simulink model "hw3_sim"  (R2022a)
settings: Solver=VariableStepAuto  StartTime=0.0  StopTime=20  RelTol=1e-3
values from neighbouring files (symbols this model uses):
  ctrl = c*K    [h3.m]
  x0 = [10 0 10 0]'    [h3.m]
settings Model: Creator=voidjocker  LastModifiedBy=voidjocker

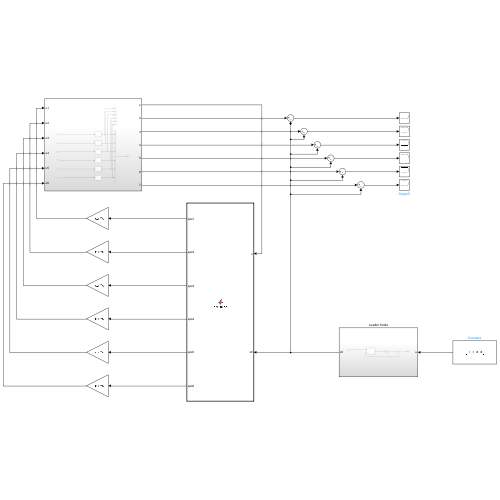
[thumbnail: Simulink's stored preview of the top-level diagram]
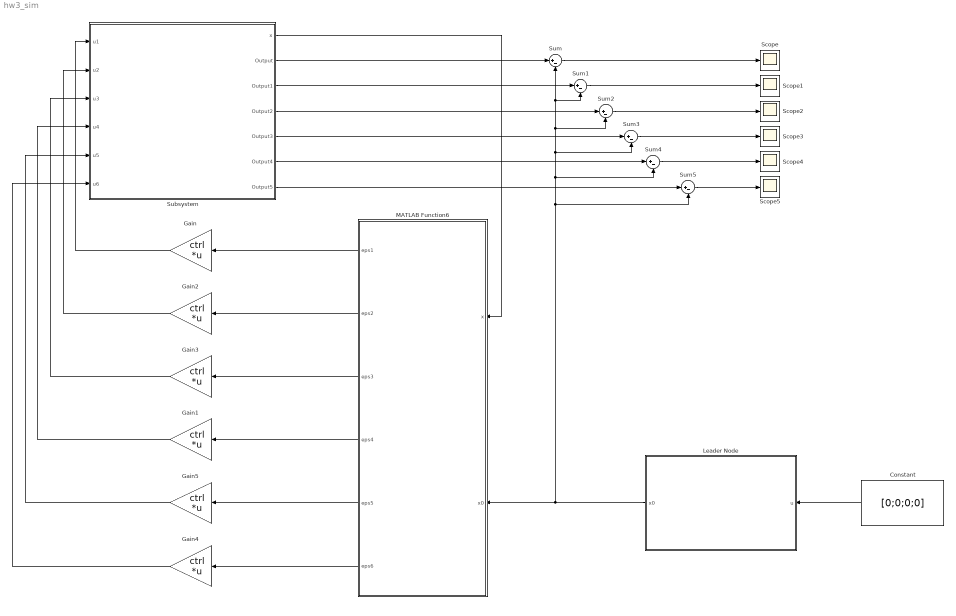
== system hw3_sim ==
  Constant : Constant  Value=[0;0;0;0]
  Gain{,1..5} (6 alike) : Gain  Gain=ctrl  Multiplication=Matrix(K*u)
  Leader Node : Subsystem
  MATLAB Function6 : MATLAB Function  TreatAsAtomicUnit=on
  Scope{,1..5} (6 alike) : Scope
  Subsystem : Subsystem
  Sum{,1..5} (6 alike) : Sum  Inputs=|+-
  wires:
  Constant/1 -> Leader Node/1(u)
  Leader Node/1(x0) -> Sum5/2, Sum4/2, Sum3/2, Sum2/2, Sum1/2, Sum/2, MATLAB Function6/2(x0)
  Subsystem/1(x) -> MATLAB Function6/1(x)
  Gain/1 -> Subsystem/1(u1)
  MATLAB Function6/1(eps1) -> Gain/1
  MATLAB Function6/2(eps2) -> Gain2/1
  MATLAB Function6/5(eps5) -> Gain5/1
  MATLAB Function6/4(eps4) -> Gain1/1
  MATLAB Function6/3(eps3) -> Gain3/1
  MATLAB Function6/6(eps6) -> Gain4/1
  Gain2/1 -> Subsystem/2(u2)
  Gain3/1 -> Subsystem/3(u3)
  Gain1/1 -> Subsystem/4(u4)
  Gain5/1 -> Subsystem/5(u5)
  Gain4/1 -> Subsystem/6(u6)
  Subsystem/2(Output) -> Sum/1
  Sum/1 -> Scope/1
  Subsystem/3(Output1) -> Sum1/1
  Subsystem/4(Output2) -> Sum2/1
  Sum2/1 -> Scope2/1
  Sum1/1 -> Scope1/1
  Sum3/1 -> Scope3/1
  Subsystem/5(Output3) -> Sum3/1
  Subsystem/6(Output4) -> Sum4/1
  Subsystem/7(Output5) -> Sum5/1
  Sum4/1 -> Scope4/1
  Sum5/1 -> Scope5/1

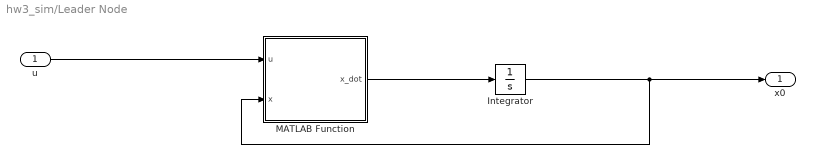
== system hw3_sim/Leader Node ==
  u : Inport
  Integrator : Integrator  InitialCondition=x0
  MATLAB Function : MATLAB Function  TreatAsAtomicUnit=on
  x0 : Outport
  wires:
  MATLAB Function/1(x_dot) -> Integrator/1
  Integrator/1 -> MATLAB Function/2(x), x0/1
  u/1 -> MATLAB Function/1(u)

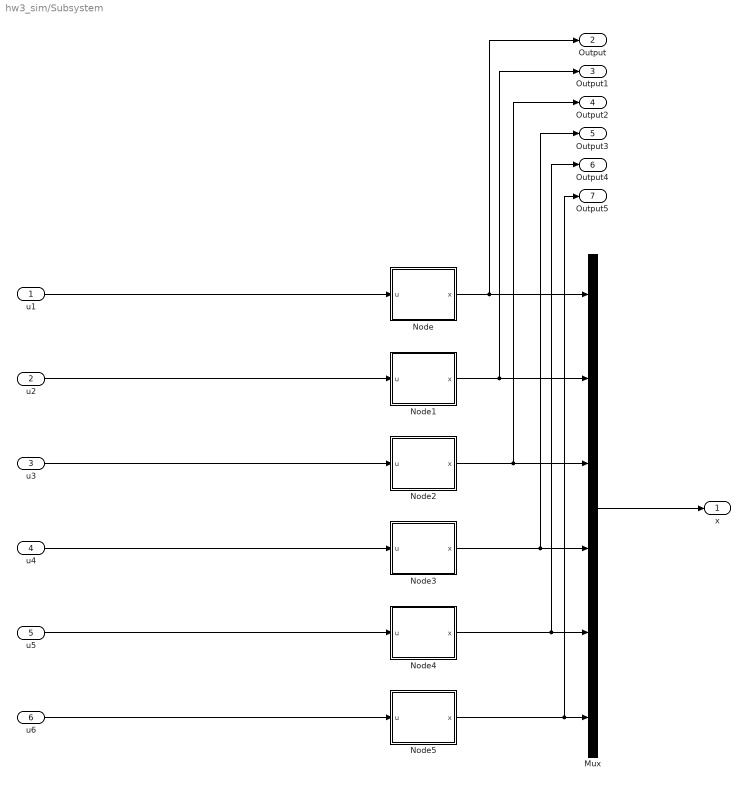
== system hw3_sim/Subsystem ==
  u1 : Inport
  u2 : Inport  Port=2
  u3 : Inport  Port=3
  u4 : Inport  Port=4
  u5 : Inport  Port=5
  u6 : Inport  Port=6
  Mux : Mux  Inputs=6
  Node : Subsystem
  Node1 : Subsystem
  Node2 : Subsystem
  Node3 : Subsystem
  Node4 : Subsystem
  Node5 : Subsystem
  x : Outport
  Output : Outport  Port=2
  Output1 : Outport  Port=3
  Output2 : Outport  Port=4
  Output3 : Outport  Port=5
  Output4 : Outport  Port=6
  Output5 : Outport  Port=7
  wires:
  Node/1(x) -> Output/1, Mux/1
  Node1/1(x) -> Output1/1, Mux/2
  Node2/1(x) -> Output2/1, Mux/3
  Node3/1(x) -> Output3/1, Mux/4
  Node4/1(x) -> Output4/1, Mux/5
  Node5/1(x) -> Output5/1, Mux/6
  Mux/1 -> x/1
  u1/1 -> Node/1(u)
  u2/1 -> Node1/1(u)
  u3/1 -> Node2/1(u)
  u4/1 -> Node3/1(u)
  u5/1 -> Node4/1(u)
  u6/1 -> Node5/1(u)

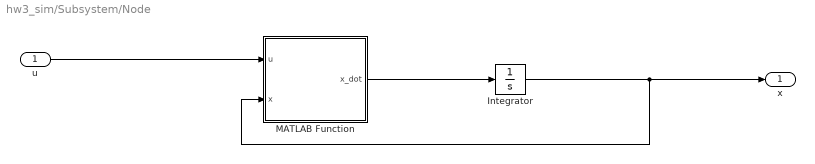
== system hw3_sim/Subsystem/Node ==
  u : Inport
  Integrator : Integrator  InitialCondition=x0
  MATLAB Function : MATLAB Function  TreatAsAtomicUnit=on
  x : Outport
  wires:
  MATLAB Function/1(x_dot) -> Integrator/1
  Integrator/1 -> MATLAB Function/2(x), x/1
  u/1 -> MATLAB Function/1(u)

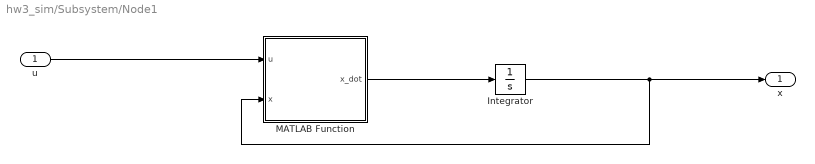
== system hw3_sim/Subsystem/Node1 ==
  u : Inport
  Integrator : Integrator  InitialCondition=x0
  MATLAB Function : MATLAB Function  TreatAsAtomicUnit=on
  x : Outport
  wires:
  MATLAB Function/1(x_dot) -> Integrator/1
  Integrator/1 -> MATLAB Function/2(x), x/1
  u/1 -> MATLAB Function/1(u)

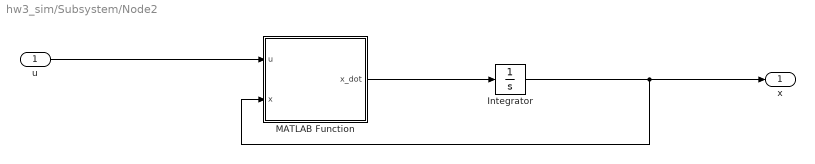
== system hw3_sim/Subsystem/Node2 ==
  u : Inport
  Integrator : Integrator  InitialCondition=x0
  MATLAB Function : MATLAB Function  TreatAsAtomicUnit=on
  x : Outport
  wires:
  MATLAB Function/1(x_dot) -> Integrator/1
  Integrator/1 -> MATLAB Function/2(x), x/1
  u/1 -> MATLAB Function/1(u)

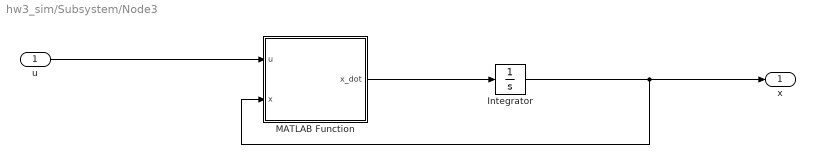
== system hw3_sim/Subsystem/Node3 ==
  u : Inport
  Integrator : Integrator  InitialCondition=x0
  MATLAB Function : MATLAB Function  TreatAsAtomicUnit=on
  x : Outport
  wires:
  MATLAB Function/1(x_dot) -> Integrator/1
  Integrator/1 -> MATLAB Function/2(x), x/1
  u/1 -> MATLAB Function/1(u)

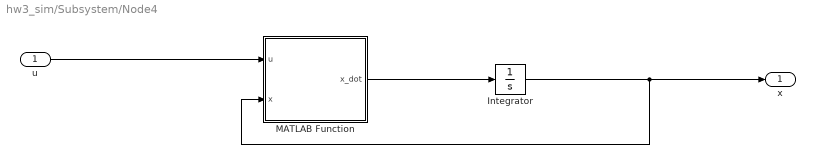
== system hw3_sim/Subsystem/Node4 ==
  u : Inport
  Integrator : Integrator  InitialCondition=x0
  MATLAB Function : MATLAB Function  TreatAsAtomicUnit=on
  x : Outport
  wires:
  MATLAB Function/1(x_dot) -> Integrator/1
  Integrator/1 -> MATLAB Function/2(x), x/1
  u/1 -> MATLAB Function/1(u)

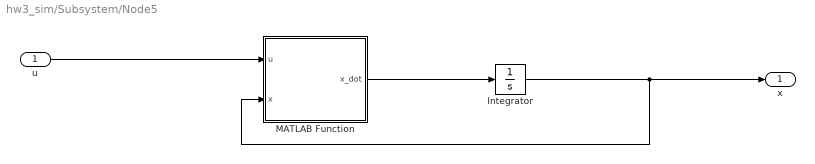
== system hw3_sim/Subsystem/Node5 ==
  u : Inport
  Integrator : Integrator  InitialCondition=x0
  MATLAB Function : MATLAB Function  TreatAsAtomicUnit=on
  x : Outport
  wires:
  MATLAB Function/1(x_dot) -> Integrator/1
  Integrator/1 -> MATLAB Function/2(x), x/1
  u/1 -> MATLAB Function/1(u)

== matlab function hw3_sim/Leader Node/MATLAB Function ==
  data: u input; x_dot output; x input
function x_dot = model(u,x)
k1 = 1.5;
k2 = 1;
m1 = 1.1;
m2 = .9;

A = [0 1 0 0
    -(k1/m1)-(k2/m1) 0 0 0
    0 0 0 1
    k2/m2 0 -k2/m2 0];

B = eye(4,4);

C = eye(4,4);

D = zeros(4,4);
x_dot = A*x + B* u;

== matlab function hw3_sim/Subsystem/Node/MATLAB Function ==
  data: u input; x_dot output; x input
function x_dot = model(u,x)
k1 = 1.5;
k2 = 1;
m1 = 1.1;
m2 = .9;
A = [0 1 0 0
    -(k1/m1)-(k2/m1) 0 0 0
    0 0 0 1
    k2/m2 0 -k2/m2 0];

B = eye(4,4);

C = eye(4,4);

D = zeros(4,4);
x_dot = A*x + B* u;

== matlab function hw3_sim/Subsystem/Node1/MATLAB Function ==
  data: u input; x_dot output; x input
function x_dot = model(u,x)
k1 = 1.5;
k2 = 1;
m1 = 1.1;
m2 = .9;

A = [0 1 0 0
    -(k1/m1)-(k2/m1) 0 0 0
    0 0 0 1
    k2/m2 0 -k2/m2 0];

B = eye(4,4);

C = eye(4,4);

D = zeros(4,4);
x_dot = A*x + B* u;

== matlab function hw3_sim/Subsystem/Node2/MATLAB Function ==
  data: u input; x_dot output; x input
function x_dot = model(u,x)
k1 = 1.5;
k2 = 1;
m1 = 1.1;
m2 = .9;

A = [0 1 0 0
    -(k1/m1)-(k2/m1) 0 0 0
    0 0 0 1
    k2/m2 0 -k2/m2 0];

B = eye(4,4);

C = eye(4,4);

D = zeros(4,4);
x_dot = A*x + B* u;

== matlab function hw3_sim/Subsystem/Node3/MATLAB Function ==
  data: u input; x_dot output; x input
function x_dot = model(u,x)
k1 = 1.5;
k2 = 1;
m1 = 1.1;
m2 = .9;

A = [0 1 0 0
    -(k1/m1)-(k2/m1) 0 0 0
    0 0 0 1
    k2/m2 0 -k2/m2 0];

B = eye(4,4);

C = eye(4,4);

D = zeros(4,4);
x_dot = A*x + B* u;

== matlab function hw3_sim/Subsystem/Node4/MATLAB Function ==
  data: u input; x_dot output; x input
function x_dot = model(u,x)
k1 = 1.5;
k2 = 1;
m1 = 1.1;
m2 = .9;

A = [0 1 0 0
    -(k1/m1)-(k2/m1) 0 0 0
    0 0 0 1
    k2/m2 0 -k2/m2 0];

B = eye(4,4);

C = eye(4,4);

D = zeros(4,4);
x_dot = A*x + B* u;

== matlab function hw3_sim/MATLAB Function6 ==
  data: x input; eps1 output; x0 input; eps2 output; eps3 output; eps4 output; eps5 output; eps6 output
function [eps1,eps2,eps3,eps4,eps5,eps6]= err_func(x,x0)

N = 6;
GM = zeros(N+1,N+1);
GM(2,1) = 1;GM(5,4) = 1;
GM(3,2) = 2;GM(6,5) = 1;
GM(4,3) = 6;GM(7,6) = 3;
g = GM(:,1);
GM = GM(2:end,1:end-1);


x = [x(1:4);x(5:8);x(9:12);x(13:16);x(17:20);x(21:24)];
eps = zeros(N,4);
for i = 1:N
    for j = 1:N
        eps(i,:) = eps(i,:) + GM(i,j)*(x(j,:)'-x(i,:)') ;
    end
    eps(i,:) = eps(i,:) + GM(i,1)*(x0'-x(i,:));
end

eps1 = eps(1,:)';
eps2 = eps(2,:)';
eps3 = eps(3,:)';
eps4 = eps(4,:)';
eps5 = eps(5,:)';
eps6 = eps(6,:)';

== matlab function hw3_sim/Subsystem/Node5/MATLAB Function ==
  data: u input; x_dot output; x input
function x_dot = model(u,x)
k1 = 1.5;
k2 = 1;
m1 = 1.1;
m2 = .9;

A = [0 1 0 0
    -(k1/m1)-(k2/m1) 0 0 0
    0 0 0 1
    k2/m2 0 -k2/m2 0];

B = eye(4,4);

C = eye(4,4);

D = zeros(4,4);
x_dot = A*x + B* u;
